simulink library "SingleWorkstationModelLibrary"  (R2014a)
settings: Solver=ode45  StartTime=0.0  StopTime=10.0  RelTol=1e-3
undefined symbols (not defined in the file or in its folder): se_randomizeseeds
(part 1 of 3)
settings Model: Creator=AnotherUser  LastModifiedBy=AnotherUser

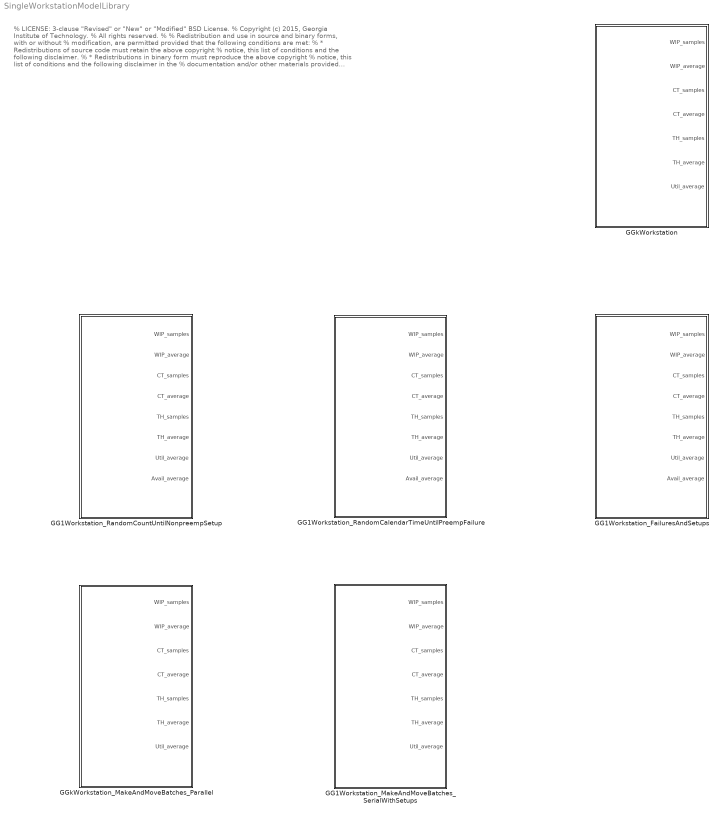
== system SingleWorkstationModelLibrary ==
  note: % LICENSE: 3-clause "Revised" or "New" or "Modified" BSD License.
      | % Copyright (c) 2015, Georgia Institute of Technology.
      | % All rights reserved.
      | %
      | % Redistribution and use in source and binary forms, with or without
      | % modification, are permitted provided that the following conditions are met:
      | % * Redistributions of source code must retain the above copyright
      | % notice, this list of conditions and the following disclaimer.
      | % * Redistributions in binary form must reproduce the above copyright
      | % notice, this list of conditions and the following disclaimer in the
      | % documentation and/or other materials provided with the distribution.
      | % * Neither the name of the Georgia Institute of Technology nor the
      | % names of its contributors may be used to endorse or promote products
      | % derived from this software without specific prior written permission.
      | %
      | % THIS SOFTWARE IS PROVIDED BY THE COPYRIGHT HOLDERS AND CONTRIBUTORS "AS IS" AND
      | % ANY EXPRESS OR IMPLIED WARRANTIES, INCLUDING, BUT NOT LIMITED TO, THE IMPLIED
      | % WARRANTIES OF MERCHANTABILITY AND FITNESS FOR A PARTICULAR PURPOSE ARE
      | % DISCLAIMED. IN NO EVENT SHALL THE GEORGIA INSTITUTE OF TECHNOLOGY BE LIABLE FOR
      | % ANY DIRECT, INDIRECT, INCIDENTAL, SPECIAL, EXEMPLARY, OR CONSEQUENTIAL DAMAGES
      | % (INCLUDING, BUT NOT LIMITED TO, PROCUREMENT OF SUBSTITUTE GOODS OR SERVICES;
      | % LOSS OF USE, DATA, OR PROFITS; OR BUSINESS INTERRUPTION) HOWEVER CAUSED AND
      | % ON ANY THEORY OF LIABILITY, WHETHER IN CONTRACT, STRICT LIABILITY, OR TORT
      | % (INCLUDING NEGLIGENCE OR OTHERWISE) ARISING IN ANY WAY OUT OF THE USE OF THIS
      | % SOFTWARE, EVEN IF ADVISED OF THE POSSIBILITY OF SUCH DAMAGE.
  GG1Workstation_FailuresAndSetups : Subsystem  InitFcn=se_randomizeseeds(gcs, 'Mode', 'All')
      settings: CopyFcn=set_param(gcb, 'LinkStatus', 'none');
  GG1Workstation_MakeAndMoveBatches_SerialWithSetups : Subsystem  InitFcn=se_randomizeseeds(gcs, 'Mode', 'All')
      settings: CopyFcn=set_param(gcb, 'LinkStatus', 'none');
  GG1Workstation_RandomCalendarTimeUntilPreempFailure : Subsystem  InitFcn=se_randomizeseeds(gcs, 'Mode', 'All')
      settings: CopyFcn=set_param(gcb, 'LinkStatus', 'none');
  GG1Workstation_RandomCountUntilNonpreempSetup : Subsystem  InitFcn=se_randomizeseeds(gcs, 'Mode', 'All')
      settings: CopyFcn=set_param(gcb, 'LinkStatus', 'none');
  GGkWorkstation : Subsystem  InitFcn=se_randomizeseeds(gcs, 'Mode', 'All')
      settings: CopyFcn=set_param(gcb, 'LinkStatus', 'none');
  GGkWorkstation_MakeAndMoveBatches_Parallel : Subsystem  InitFcn=se_randomizeseeds(gcs, 'Mode', 'All')
      settings: CopyFcn=set_param(gcb, 'LinkStatus', 'none');

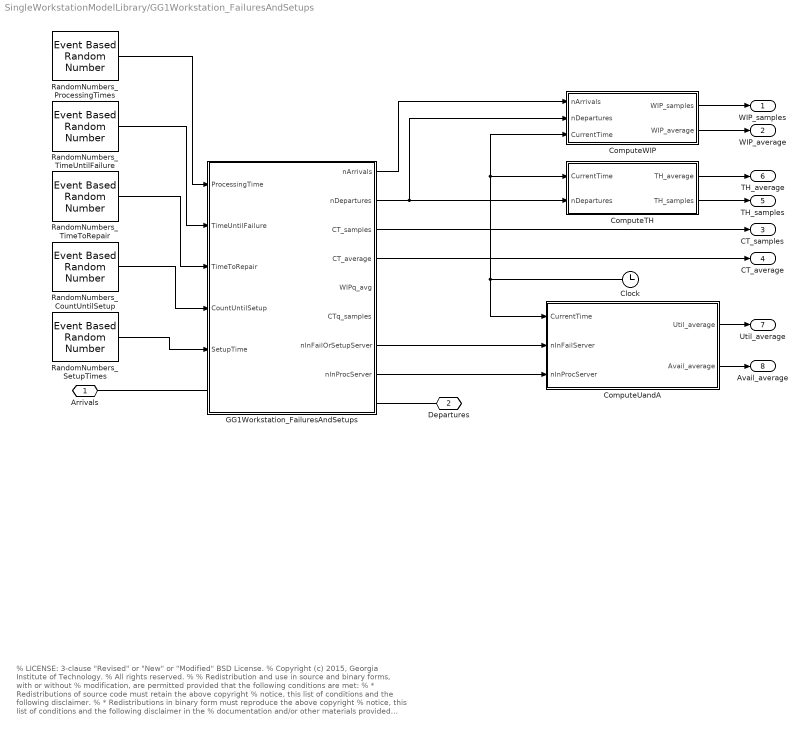
== system SingleWorkstationModelLibrary/GG1Workstation_FailuresAndSetups ==
  note: % LICENSE: 3-clause "Revised" or "New" or "Modified" BSD License.
      | % Copyright (c) 2015, Georgia Institute of Technology.
      | % All rights reserved.
      | %
      | % Redistribution and use in source and binary forms, with or without
      | % modification, are permitted provided that the following conditions are met:
      | % * Redistributions of source code must retain the above copyright
      | % notice, this list of conditions and the following disclaimer.
      | % * Redistributions in binary form must reproduce the above copyright
      | % notice, this list of conditions and the following disclaimer in the
      | % documentation and/or other materials provided with the distribution.
      | % * Neither the name of the Georgia Institute of Technology nor the
      | % names of its contributors may be used to endorse or promote products
      | % derived from this software without specific prior written permission.
      | %
      | % THIS SOFTWARE IS PROVIDED BY THE COPYRIGHT HOLDERS AND CONTRIBUTORS "AS IS" AND
      | % ANY EXPRESS OR IMPLIED WARRANTIES, INCLUDING, BUT NOT LIMITED TO, THE IMPLIED
      | % WARRANTIES OF MERCHANTABILITY AND FITNESS FOR A PARTICULAR PURPOSE ARE
      | % DISCLAIMED. IN NO EVENT SHALL THE GEORGIA INSTITUTE OF TECHNOLOGY BE LIABLE FOR
      | % ANY DIRECT, INDIRECT, INCIDENTAL, SPECIAL, EXEMPLARY, OR CONSEQUENTIAL DAMAGES
      | % (INCLUDING, BUT NOT LIMITED TO, PROCUREMENT OF SUBSTITUTE GOODS OR SERVICES;
      | % LOSS OF USE, DATA, OR PROFITS; OR BUSINESS INTERRUPTION) HOWEVER CAUSED AND
      | % ON ANY THEORY OF LIABILITY, WHETHER IN CONTRACT, STRICT LIABILITY, OR TORT
      | % (INCLUDING NEGLIGENCE OR OTHERWISE) ARISING IN ANY WAY OUT OF THE USE OF THIS
      | % SOFTWARE, EVEN IF ADVISED OF THE POSSIBILITY OF SUCH DAMAGE.
  Clock : Clock
  ComputeTH : Subsystem
  ComputeUandA : Subsystem
  ComputeWIP : Subsystem
  GG1Workstation_FailuresAndSetups : Subsystem  mask{Capacity=Inf}
      mask prompts: Capacity "Queue Capacity"
      mask TypeOptions Capacity: FIFOQueue/Capacity
      mask DialogControl DescTextVar Prompt: GG1 Workstation, with a random count of entities serviced until a setup, and random setup times.  Setups are functionally equivalent to any non-preemptive (e.g. non-interrupting) downtime, for example preventative maintenance.
  RandomNumbers_CountUntilSetup : EventBasedRandomNumber  meanExp=100  minUnif=40  maxUnif=40  pOneBern=40  pSuccessBino=40  numTrialBino=40  minTri=10  maxTri=10  modeTri=10  scaleGam=166.6667  shapeGam=0.72  meanNorm=200  stdNorm=eps  pSuccessGeo=40  meanPoiss=40  thresholdLogn=40  scaleLogn=40  shapeLogn=40  thresholdLogl=40  scaleLogl=40  minBeta=40  maxBeta=40  shape1Beta=40  shape2Beta=40  minUnid=40  maxUnid=40  numValueUnid=40  thresholdWbl=40  scaleWbl=40  shapeWbl=40  valueVecCont=40  cdfVecCont=40  valueVecDisc=40  probVecDisc=40  Seed=13103
  RandomNumbers_ProcessingTimes : EventBasedRandomNumber  meanExp=75  minUnif=40  maxUnif=40  pOneBern=40  pSuccessBino=40  numTrialBino=40  minTri=40  maxTri=40  modeTri=40  thresholdGam=40  scaleGam=40  shapeGam=40  meanNorm=50  stdNorm=eps  pSuccessGeo=40  meanPoiss=40  thresholdLogn=40  scaleLogn=40  shapeLogn=40  thresholdLogl=40  scaleLogl=40  minBeta=40  maxBeta=40  shape1Beta=40  shape2Beta=40  minUnid=40  maxUnid=40  numValueUnid=40  thresholdWbl=40  scaleWbl=40  shapeWbl=40  valueVecCont=40  cdfVecCont=40  valueVecDisc=40  probVecDisc=40  Seed=16319
  RandomNumbers_SetupTimes : EventBasedRandomNumber  meanExp=400  minUnif=40  maxUnif=40  pOneBern=40  pSuccessBino=40  numTrialBino=40  minTri=38  maxTri=38  modeTri=38  scaleGam=20  meanNorm=200  stdNorm=eps  pSuccessGeo=40  meanPoiss=40  thresholdLogn=40  scaleLogn=40  shapeLogn=40  thresholdLogl=40  scaleLogl=40  minBeta=40  maxBeta=40  shape1Beta=40  shape2Beta=40  minUnid=40  maxUnid=40  numValueUnid=40  thresholdWbl=40  scaleWbl=40  shapeWbl=40  valueVecCont=40  cdfVecCont=40  probVecDisc=[0 1]  Seed=19536
  RandomNumbers_TimeToRepair : EventBasedRandomNumber  meanExp=400  minUnif=40  maxUnif=40  pOneBern=40  pSuccessBino=40  numTrialBino=40  minTri=38  maxTri=38  modeTri=38  scaleGam=20  meanNorm=400  stdNorm=eps  pSuccessGeo=40  meanPoiss=40  thresholdLogn=40  scaleLogn=40  shapeLogn=40  thresholdLogl=40  scaleLogl=40  minBeta=40  maxBeta=40  shape1Beta=40  shape2Beta=40  minUnid=40  maxUnid=40  numValueUnid=40  thresholdWbl=40  scaleWbl=40  shapeWbl=40  valueVecCont=40  cdfVecCont=40  probVecDisc=[0 1]  Seed=22753
  RandomNumbers_TimeUntilFailure : EventBasedRandomNumber  meanExp=2500  minUnif=40  maxUnif=40  pOneBern=40  pSuccessBino=40  numTrialBino=40  minTri=114  maxTri=114  modeTri=114  scaleGam=166.6667  shapeGam=0.72  meanNorm=2000  stdNorm=eps  pSuccessGeo=40  meanPoiss=40  thresholdLogn=40  scaleLogn=40  shapeLogn=40  thresholdLogl=40  scaleLogl=40  minBeta=40  maxBeta=40  shape1Beta=40  shape2Beta=40  minUnid=40  maxUnid=40  numValueUnid=40  thresholdWbl=40  scaleWbl=40  shapeWbl=40  valueVecCont=40  cdfVecCont=40  valueVecDisc=40  probVecDisc=40  Seed=25970
  Arrivals : PMIOPort  Port=1  Side=Left
  Departures : PMIOPort  Port=2  Side=Right
  WIP_samples : Outport
  WIP_average : Outport  Port=2
  CT_samples : Outport  Port=3
  CT_average : Outport  Port=4
  TH_samples : Outport  Port=5
  TH_average : Outport  Port=6
  Util_average : Outport  Port=7
  Avail_average : Outport  Port=8
  wires:
  RandomNumbers_ProcessingTimes/1 -> GG1Workstation_FailuresAndSetups/1(ProcessingTime)
  GG1Workstation_FailuresAndSetups/2(nDepartures) -> ComputeWIP/2(nDepartures), ComputeTH/2(nDepartures)
  GG1Workstation_FailuresAndSetups/3(CT_samples) -> CT_samples/1
  GG1Workstation_FailuresAndSetups/4(CT_average) -> CT_average/1
  ComputeWIP/1(WIP_samples) -> WIP_samples/1
  ComputeWIP/2(WIP_average) -> WIP_average/1
  GG1Workstation_FailuresAndSetups/1(nArrivals) -> ComputeWIP/1(nArrivals)
  Clock/1 -> ComputeWIP/3(CurrentTime), ComputeTH/1(CurrentTime), ComputeUandA/1(CurrentTime)
  ComputeTH/1(TH_average) -> TH_average/1
  ComputeTH/2(TH_samples) -> TH_samples/1
  RandomNumbers_TimeUntilFailure/1 -> GG1Workstation_FailuresAndSetups/2(TimeUntilFailure)
  RandomNumbers_TimeToRepair/1 -> GG1Workstation_FailuresAndSetups/3(TimeToRepair)
  RandomNumbers_CountUntilSetup/1 -> GG1Workstation_FailuresAndSetups/4(CountUntilSetup)
  RandomNumbers_SetupTimes/1 -> GG1Workstation_FailuresAndSetups/5(SetupTime)
  GG1Workstation_FailuresAndSetups/7(nInFailOrSetupServer) -> ComputeUandA/2(nInFailServer)
  GG1Workstation_FailuresAndSetups/8(nInProcServer) -> ComputeUandA/3(nInProcServer)
  ComputeUandA/1(Util_average) -> Util_average/1
  ComputeUandA/2(Avail_average) -> Avail_average/1
  connections:
  GG1Workstation_FailuresAndSetups/RConn1 -- Departures/RConn1
  Arrivals/RConn1 -- GG1Workstation_FailuresAndSetups/LConn1

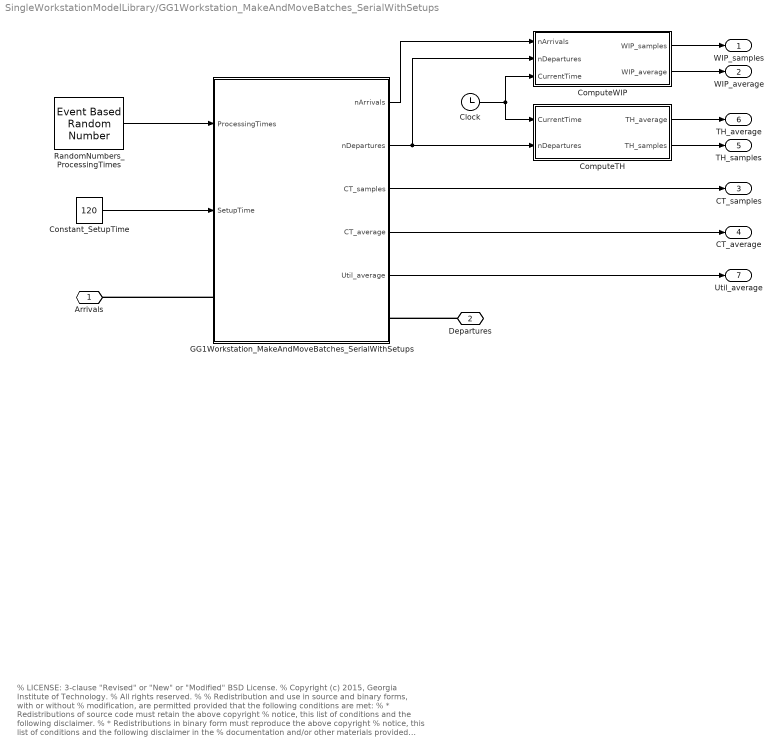
== system SingleWorkstationModelLibrary/GG1Workstation_MakeAndMoveBatches_SerialWithSetups ==
  note: % LICENSE: 3-clause "Revised" or "New" or "Modified" BSD License.
      | % Copyright (c) 2015, Georgia Institute of Technology.
      | % All rights reserved.
      | %
      | % Redistribution and use in source and binary forms, with or without
      | % modification, are permitted provided that the following conditions are met:
      | % * Redistributions of source code must retain the above copyright
      | % notice, this list of conditions and the following disclaimer.
      | % * Redistributions in binary form must reproduce the above copyright
      | % notice, this list of conditions and the following disclaimer in the
      | % documentation and/or other materials provided with the distribution.
      | % * Neither the name of the Georgia Institute of Technology nor the
      | % names of its contributors may be used to endorse or promote products
      | % derived from this software without specific prior written permission.
      | %
      | % THIS SOFTWARE IS PROVIDED BY THE COPYRIGHT HOLDERS AND CONTRIBUTORS "AS IS" AND
      | % ANY EXPRESS OR IMPLIED WARRANTIES, INCLUDING, BUT NOT LIMITED TO, THE IMPLIED
      | % WARRANTIES OF MERCHANTABILITY AND FITNESS FOR A PARTICULAR PURPOSE ARE
      | % DISCLAIMED. IN NO EVENT SHALL THE GEORGIA INSTITUTE OF TECHNOLOGY BE LIABLE FOR
      | % ANY DIRECT, INDIRECT, INCIDENTAL, SPECIAL, EXEMPLARY, OR CONSEQUENTIAL DAMAGES
      | % (INCLUDING, BUT NOT LIMITED TO, PROCUREMENT OF SUBSTITUTE GOODS OR SERVICES;
      | % LOSS OF USE, DATA, OR PROFITS; OR BUSINESS INTERRUPTION) HOWEVER CAUSED AND
      | % ON ANY THEORY OF LIABILITY, WHETHER IN CONTRACT, STRICT LIABILITY, OR TORT
      | % (INCLUDING NEGLIGENCE OR OTHERWISE) ARISING IN ANY WAY OUT OF THE USE OF THIS
      | % SOFTWARE, EVEN IF ADVISED OF THE POSSIBILITY OF SUCH DAMAGE.
  Clock : Clock
  ComputeTH : Subsystem
  ComputeWIP : Subsystem
  Constant_SetupTime : Constant  Value=120
  GG1Workstation_MakeAndMoveBatches_SerialWithSetups : Subsystem  mask{MakeBatchSize=10, MoveBatchSize=1}
      mask prompts: MakeBatchSize "Make (a.k.a. Process) Batch Size:"; MoveBatchSize "Move (a.k.a. Transfer) Batch Size"
      mask Callback MakeBatchSize:
      | %% Capture pre-existing base workspace variables, to cleanup when done
      | preExistingVars = who;
      | 
      | 
      | %% MakeBatchSize is defined as a mask parameter
      | batchSizeStr = get_param(gcbh, 'MakeBatchSize');
      | batchSizeInt = int32(str2double(batchSizeStr));  %Enforce integer
      | if batchSizeInt < 1  %str2double returns NaN for non-numerical input, and int32 returns 0 for NaN
      |     error('Invalid input for MakeBatchSize');
      | end
      | set_param(gcbh, 'MakeBatchSize', num2str(batchSizeInt));  %Correct any non-integer value
      | 
      | 
      | %% Get paths of OutputSwitch, EntityCombiner, EntitySplitter, and PathCombiner
      | singleWksPath = [gcs '/' get(gcbh,'Name')];
      | outputSwitchPath = [singleWksPath '/MakeBatchOutputSwitch'];
      | entityCombinerPath = [singleWksPath '/MakeBatchEntityCombiner'];
      | entitySplitterPath = [singleWksPath '/MakeBatchEntitySplitter'];
      | pathCombinerPath = [singleWksPath '/MakeBatchPathCombiner'];
      | 
      | 
      | %% NEW
      | constantPath = [singleWksPath '/Constant_MakeBatchSize'];
      | set_param(constantPath, 'Value', num2str(batchSizeInt));
      | 
      | 
      | %% Unsure if needed:  Disable model library link to enable editing
      | %set_param(singleWksPath, 'LinkStatus', 'inactive');
      | 
      | 
      | %% Delete existing queues and connections
      | phOutputSwitch = get_param(outputSwitchPath, 'PortHandles');
      | phOutputSwitch = phOutputSwitch.RConn;
      | phEntityCombiner = get_param(entityCombinerPath, 'PortHandles');
      | phEntityCombiner = phEntityCombiner.LConn;
      | phEntitySplitter = get_param(entitySplitterPath, 'PortHandles');
      | phEntitySplitter = phEntitySplitter.RConn;
      | phPathCombiner = get_param(pathCombinerPath, 'PortHandles');
      | phPathCombiner = phPathCombiner.LConn;
      | 
      | 
      | %Delete existing queues
      | oldBatchSize = get_param(outputSwitchPath, 'NumberOutputPorts');
      | queueNamesBeginWith = 'MakeBatchQ';  %Hard-codes a particular naming scheme
      | singleWksBlockList = get(gcbh, 'Blocks');
      | ECQueueMatches = strncmpi(queueNamesBeginWith, singleWksBlockList, length(queueNamesBeginWith));
      | ECQueueNames = singleWksBlockList(ECQueueMatches);
      | if ~isempty(ECQueueNames)
      |     for mmmmm = 1 : length(ECQueueNames)
      |         queuePath = [singleWksPath '/' ECQueueNames{mmmmm}];
      |         queueHandle = get_param(queuePath, 'Handle');
      |         delete(queueHandle);
      |     end
      | end
      | 
      | %Delete the lines
      | for iiiii = 1 : str2double(oldBatchSize)
      |     phOutputSwitchPos = get_param(phOutputSwitch(iiiii), 'Position');
      |     try delete_line(singleWksPath, phOutputSwitchPos); catch, end  %Fail silently
      |     phEntityCombinerPos = get_param(phEntityCombiner(iiiii), 'Position');
      |     try delete_line(singleWksPath, phEntityCombinerPos); catch, end  %Fail silently
      |     phEntitySplitterPos = get_param(phEntitySplitter(iiiii), 'Position');
      |     try delete_line(singleWksPath, phEntitySplitterPos); catch, end  %Fail silently
      | 	phPathCombinerPos = get_param(phPathCombiner(iiiii), 'Position');
      | 	try delete_line(singleWksPath, phPathCombinerPos); catch, end  %Fail silently
      | end
      | 
      | 
      | %% Set new number of ports
      | set_param(outputSwitchPath, 'NumberOutputPorts', batchSizeStr);
      | set_param(entityCombinerPath, 'NumberInputPorts', batchSizeStr);
      | set_param(entitySplitterPath, 'NumberOutputPorts', batchSizeStr);
      | set_param(pathCombinerPath, 'NumberInputPorts', batchSizeStr);
      | 
      | 
      | %% Add queues and connectors
      | phOutputSwitch = get_param(outputSwitchPath, 'PortHandles');
      | phOutputSwitch = phOutputSwitch.RConn;
      | phEntityCombiner = get_param(entityCombinerPath, 'PortHandles');
      | phEntityCombiner = phEntityCombiner.LConn;
      | phEntitySplitter = get_param(entitySplitterPath, 'PortHandles');
      | phEntitySplitter = phEntitySplitter.RConn;
      | phPathCombiner = get_param(pathCombinerPath, 'PortHandles');
      | phPathCombiner = phPathCombiner.LConn;
      | 
      | queueLength = 80;
      | queueHeight = 20;
      | xOffset = 130;
      | prevBlockPos1 = get_param(outputSwitchPath, 'Position');
      | prevBlockPos2 = get_param(entitySplitterPath, 'Position');
      | prevBlockHeight1 = prevBlockPos1(4)-prevBlockPos1(2);
      | prevBlockHeight2 = prevBlockPos2(4)-prevBlockPos2(2);
      | yIncrement1 = prevBlockHeight1 / batchSizeInt;
      | yIncrement2 = prevBlockHeight2 / batchSizeInt;
      | for jjjjj = 1 : batchSizeInt
      | 	%%%%%%%%%%
      | 	%OutputSwitch to EntityCombiner
      |     queuePath = [singleWksPath '/' queueNamesBeginWith num2str(jjjjj) 'a'];
      |     queueHandle = add_block('built-in/FIFOQueue', queuePath);
      |     set_param(queueHandle, 'Capacity', 'Inf');  %Shouldn't be needed, but a good default
      | 
      |     left = prevBlockPos1(1)+xOffset;
      |     top = double( prevBlockPos1(2)+(jjjjj-1)*yIncrement1 );
      |     right = prevBlockPos1(1)+xOffset+queueLength;
      |     bottom = double( prevBlockPos1(2)+(jjjjj-1)*yIncrement1+queueHeight );
      |     p = [left top right bottom];
      |     set_param(queueHandle, 'Position', p);  %Need a vector of doubles (not int32)
      | 
      |     QueuePortHandles = get_param(queueHandle, 'PortHandles');
      |     %Line from OutputSwitch to Queue
      |     OutputSwitchOutPortPos = get_param(phOutputSwitch(jjjjj), 'Position');
      |     QueueInPortPos = get_param(QueuePortHandles.LConn, 'Position');
      |     add_line(singleWksPath, [OutputSwitchOutPortPos; QueueInPortPos]);
      |     %Line from Queue to EntityCombiner
      |     QueueOutPortPos = get_param(QueuePortHandles.RConn, 'Position');
      |     EntityCombinerInPortPos = get_param(phEntityCombiner(jjjjj), 'Position');
      |     add_line(singleWksPath, [QueueOutPortPos; EntityCombinerInPortPos]);
      | 
      | 	%%%%%%%%%%
      | 	%EntitySplitter to PathCombiner
      | 	queuePath = [singleWksPath '/' queueNamesBeginWith num2str(jjjjj) 'b'];
      |     queueHandle = add_block('built-in/FIFOQueue', queuePath);
      |     set_param(queueHandle, 'Capacity', num2str(1));  %Second set of queues have capacity 1
      | 
      |     left = prevBlockPos2(1)+xOffset;
      |     top = double( prevBlockPos2(2)+(jjjjj-1)*yIncrement2 );
      |     right = prevBlockPos2(1)+xOffset+queueLength;
      |     bottom = double( prevBlockPos2(2)+(jjjjj-1)*yIncrement2+queueHeight );
      |     p = [left top right bottom];
      |     set_param(queueHandle, 'Position', p);  %Need a vector of doubles (not int32)
      | 
      |     QueuePortHandles = get_param(queueHandle, 'PortHandles');
      |     %Line from OutputSwitch to Queue
      |     EntitySplitterOutPortPos = get_param(phEntitySplitter(jjjjj), 'Position');
      |     QueueInPortPos = get_param(QueuePortHandles.LConn, 'Position');
      |     add_line(singleWksPath, [EntitySplitterOutPortPos; QueueInPortPos]);
      |     %Line from Queue to EntityCombiner
      |     QueueOutPortPos = get_param(QueuePortHandles.RConn, 'Position');
      |     PathCombinerInPortPos = get_param(phPathCombiner(jjjjj), 'Position');
      |     add_line(singleWksPath, [QueueOutPortPos; PathCombinerInPortPos ]);
      | end
      | 
      | 
      | %% Cleanup, because mask callback executes in base workspace
      | clearvars('-except', preExistingVars{:});
      mask Callback MoveBatchSize:
      | %% Capture pre-existing base workspace variables, to cleanup when done
      | preExistingVars = who;
      | 
      | 
      | %% MoveBatchSize is defined as a mask parameter
      | batchSizeStr = get_param(gcbh, 'MoveBatchSize');
      | batchSizeInt = int32(str2double(batchSizeStr));  %Enforce integer
      | if batchSizeInt < 1  %str2double returns NaN for non-numerical input, and int32 returns 0 for NaN
      |     error('Invalid input for MoveBatchSize');
      | end
      | set_param(gcbh, 'MoveBatchSize', num2str(batchSizeInt));  %Correct any non-integer value
      | 
      | 
      | %% Get paths of OutputSwitch, EntityCombiner, EntitySplitter, and PathCombiner
      | singleWksPath = [gcs '/' get(gcbh,'Name')];
      | outputSwitchPath = [singleWksPath '/MoveBatchOutputSwitch'];
      | entityCombinerPath = [singleWksPath '/MoveBatchEntityCombiner'];
      | entitySplitterPath = [singleWksPath '/MoveBatchEntitySplitter'];
      | pathCombinerPath = [singleWksPath '/MoveBatchPathCombiner'];
      | 
      | 
      | %% Unsure if needed:  Disable model library link to enable editing
      | %set_param(singleWksPath, 'LinkStatus', 'inactive');
      | 
      | 
      | %% Delete existing queues and connections
      | phOutputSwitch = get_param(outputSwitchPath, 'PortHandles');
      | phOutputSwitch = phOutputSwitch.RConn;
      | phEntityCombiner = get_param(entityCombinerPath, 'PortHandles');
      | phEntityCombiner = phEntityCombiner.LConn;
      | phEntitySplitter = get_param(entitySplitterPath, 'PortHandles');
      | phEntitySplitter = phEntitySplitter.RConn;
      | 
      | %Delete existing queues
      | oldBatchSize = get_param(outputSwitchPath, 'NumberOutputPorts');
      | queueNamesBeginWith = 'MoveBatchQ';  %Hard-codes a particular naming scheme
      | singleWksBlockList = get(gcbh, 'Blocks');
      | ECQueueMatches = strncmpi(queueNamesBeginWith, singleWksBlockList, length(queueNamesBeginWith));
      | ECQueueNames = singleWksBlockList(ECQueueMatches);
      | if ~isempty(ECQueueNames)
      |     for mmmmm = 1 : length(ECQueueNames)
      |         queuePath = [singleWksPath '/' ECQueueNames{mmmmm}];
      |         queueHandle = get_param(queuePath, 'Handle');
      |         delete(queueHandle);
      |     end
      | end
      | 
      | %Delete the lines
      | for iiiii = 1 : str2double(oldBatchSize)
      |     phOutputSwitchPos = get_param(phOutputSwitch(iiiii), 'Position');
      |     try delete_line(singleWksPath, phOutputSwitchPos); catch, end  %Fail silently
      |     phEntityCombinerPos = get_param(phEntityCombiner(iiiii), 'Position');
      |     try delete_line(singleWksPath, phEntityCombinerPos); catch, end  %Fail silently
      |     phEntitySplitterPos = get_param(phEntitySplitter(iiiii), 'Position');
      |     try delete_line(singleWksPath, phEntitySplitterPos); catch, end  %Fail silently
      | end
      | 
      | 
      | %% Set new number of ports
      | set_param(outputSwitchPath, 'NumberOutputPorts', batchSizeStr);
      | set_param(entityCombinerPath, 'NumberInputPorts', batchSizeStr);
      | set_param(entitySplitterPath, 'NumberOutputPorts', batchSizeStr);
      | set_param(pathCombinerPath, 'NumberInputPorts', batchSizeStr);
      | 
      | 
      | %% Add EntityCombiner input queues, plus connections between OutputSwitch and EntityCombiner
      | phOutputSwitch = get_param(outputSwitchPath, 'PortHandles');
      | phOutputSwitch = phOutputSwitch.RConn;
      | phEntityCombiner = get_param(entityCombinerPath, 'PortHandles');
      | phEntityCombiner = phEntityCombiner.LConn;
      | phEntitySplitter = get_param(entitySplitterPath, 'PortHandles');
      | phEntitySplitter = phEntitySplitter.RConn;
      | phPathCombiner = get_param(pathCombinerPath, 'PortHandles');
      | phPathCombiner = phPathCombiner.LConn;
      | 
      | queueLength = 80;
      | queueHeight = 20;
      | xOffset = 130;
      | prevBlockPos = get_param(outputSwitchPath, 'Position');
      | prevBlockHeight = prevBlockPos(4)-prevBlockPos(2);
      | yIncrement = prevBlockHeight / batchSizeInt;
      | for jjjjj = 1 : batchSizeInt
      |     queuePath = [singleWksPath '/' queueNamesBeginWith num2str(jjjjj)];
      |     queueHandle = add_block('built-in/FIFOQueue', queuePath);
      |     set_param(queueHandle, 'Capacity', '1');
      | 
      | 	left = prevBlockPos(1)+xOffset;
      |     top = double( prevBlockPos(2)+(jjjjj-1)*yIncrement );
      |     right = prevBlockPos(1)+xOffset+queueLength;
      |     bottom = double( prevBlockPos(2)+(jjjjj-1)*yIncrement+queueHeight );
      |     p = [left top right bottom];
      |     set_param(queueHandle, 'Position', p);  %Need a vector of doubles (not int32)
      | 
      |     QueuePortHandles = get_param(queueHandle, 'PortHandles');
      |     %Line from OutputSwitch to Queue
      |     OutputSwitchOutPortPos = get_param(phOutputSwitch(jjjjj), 'Position');
      |     QueueInPortPos = get_param(QueuePortHandles.LConn, 'Position');
      |     add_line(singleWksPath, [OutputSwitchOutPortPos; QueueInPortPos]);
      |     %Line from Queue to EntityCombiner
      |     QueueOutPortPos = get_param(QueuePortHandles.RConn, 'Position');
      |     EntityCombinerInPortPos = get_param(phEntityCombiner(jjjjj), 'Position');
      |     add_line(singleWksPath, [QueueOutPortPos; EntityCombinerInPortPos]);
      | end
      | 
      | 
      | %% Add connections between EntitySplitter and PathCombiner
      | for kkkkk = 1 : batchSizeInt
      |     phEntitySplitterPos = get_param(phEntitySplitter(kkkkk), 'Position');
      |     phPathCombinerPos = get_param(phPathCombiner(kkkkk), 'Position');
      |     add_line(singleWksPath, [phEntitySplitterPos; phPathCombinerPos]);
      | end
      | 
      | 
      | %% Cleanup, because mask callback executes in base workspace
      | clearvars('-except', preExistingVars{:});
      mask DialogControl DescTextVar Prompt: GGk Workstation with Make and Move Batches.  This model implements serial batch processing, meaning Processing Time is for each element in a make (a.k.a. process) batch.  Tokens are output only after a full move (a.k.a. transfer) batch is assembled, and are output individually (as individual entities, not as a batch entity).
  RandomNumbers_ProcessingTimes : EventBasedRandomNumber  Distribution=Gaussian (normal)  meanExp=10  minUnif=40  maxUnif=40  pOneBern=40  pSuccessBino=40  numTrialBino=40  minTri=40  maxTri=40  modeTri=40  thresholdGam=40  scaleGam=40  shapeGam=40  meanNorm=10  stdNorm=eps  pSuccessGeo=40  meanPoiss=40  thresholdLogn=40  scaleLogn=40  shapeLogn=40  thresholdLogl=40  scaleLogl=40  minBeta=40  maxBeta=40  shape1Beta=40  shape2Beta=40  minUnid=40  maxUnid=40  numValueUnid=40  thresholdWbl=40  scaleWbl=40  shapeWbl=40  valueVecCont=40  cdfVecCont=40  valueVecDisc=40  probVecDisc=40  Seed=54923
  Arrivals : PMIOPort  Port=1  Side=Left
  Departures : PMIOPort  Port=2  Side=Right
  WIP_samples : Outport
  WIP_average : Outport  Port=2
  CT_samples : Outport  Port=3
  CT_average : Outport  Port=4
  TH_samples : Outport  Port=5
  TH_average : Outport  Port=6
  Util_average : Outport  Port=7
  wires:
  RandomNumbers_ProcessingTimes/1 -> GG1Workstation_MakeAndMoveBatches_SerialWithSetups/1(ProcessingTimes)
  GG1Workstation_MakeAndMoveBatches_SerialWithSetups/2(nDepartures) -> ComputeWIP/2(nDepartures), ComputeTH/2(nDepartures)
  GG1Workstation_MakeAndMoveBatches_SerialWithSetups/3(CT_samples) -> CT_samples/1
  GG1Workstation_MakeAndMoveBatches_SerialWithSetups/4(CT_average) -> CT_average/1
  ComputeWIP/1(WIP_samples) -> WIP_samples/1
  ComputeWIP/2(WIP_average) -> WIP_average/1
  GG1Workstation_MakeAndMoveBatches_SerialWithSetups/1(nArrivals) -> ComputeWIP/1(nArrivals)
  Clock/1 -> ComputeTH/1(CurrentTime), ComputeWIP/3(CurrentTime)
  ComputeTH/1(TH_average) -> TH_average/1
  ComputeTH/2(TH_samples) -> TH_samples/1
  GG1Workstation_MakeAndMoveBatches_SerialWithSetups/5(Util_average) -> Util_average/1
  Constant_SetupTime/1 -> GG1Workstation_MakeAndMoveBatches_SerialWithSetups/2(SetupTime)
  connections:
  Departures/RConn1 -- GG1Workstation_MakeAndMoveBatches_SerialWithSetups/RConn1
  GG1Workstation_MakeAndMoveBatches_SerialWithSetups/LConn1 -- Arrivals/RConn1

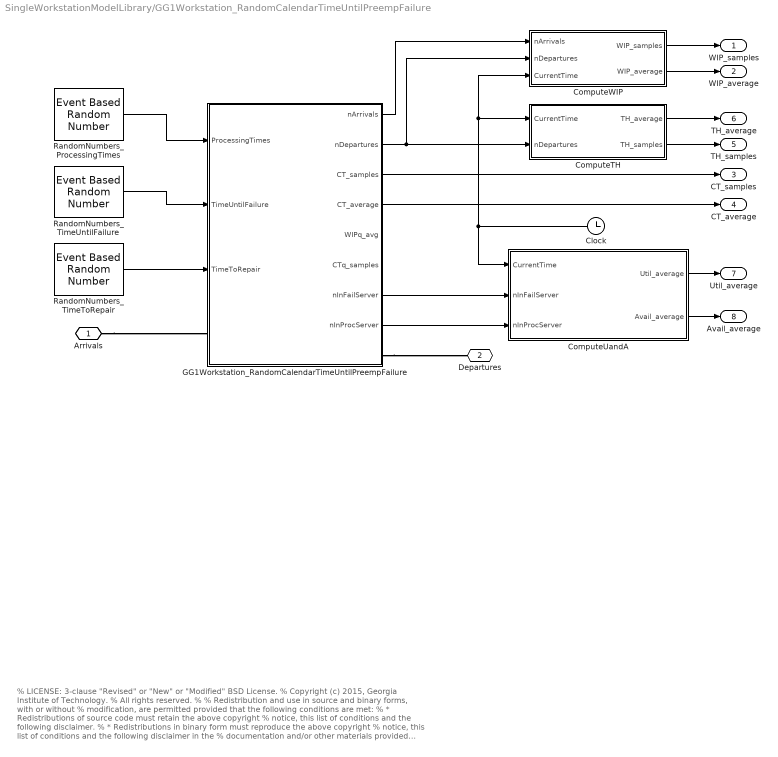
== system SingleWorkstationModelLibrary/GG1Workstation_RandomCalendarTimeUntilPreempFailure ==
  note: % LICENSE: 3-clause "Revised" or "New" or "Modified" BSD License.
      | % Copyright (c) 2015, Georgia Institute of Technology.
      | % All rights reserved.
      | %
      | % Redistribution and use in source and binary forms, with or without
      | % modification, are permitted provided that the following conditions are met:
      | % * Redistributions of source code must retain the above copyright
      | % notice, this list of conditions and the following disclaimer.
      | % * Redistributions in binary form must reproduce the above copyright
      | % notice, this list of conditions and the following disclaimer in the
      | % documentation and/or other materials provided with the distribution.
      | % * Neither the name of the Georgia Institute of Technology nor the
      | % names of its contributors may be used to endorse or promote products
      | % derived from this software without specific prior written permission.
      | %
      | % THIS SOFTWARE IS PROVIDED BY THE COPYRIGHT HOLDERS AND CONTRIBUTORS "AS IS" AND
      | % ANY EXPRESS OR IMPLIED WARRANTIES, INCLUDING, BUT NOT LIMITED TO, THE IMPLIED
      | % WARRANTIES OF MERCHANTABILITY AND FITNESS FOR A PARTICULAR PURPOSE ARE
      | % DISCLAIMED. IN NO EVENT SHALL THE GEORGIA INSTITUTE OF TECHNOLOGY BE LIABLE FOR
      | % ANY DIRECT, INDIRECT, INCIDENTAL, SPECIAL, EXEMPLARY, OR CONSEQUENTIAL DAMAGES
      | % (INCLUDING, BUT NOT LIMITED TO, PROCUREMENT OF SUBSTITUTE GOODS OR SERVICES;
      | % LOSS OF USE, DATA, OR PROFITS; OR BUSINESS INTERRUPTION) HOWEVER CAUSED AND
      | % ON ANY THEORY OF LIABILITY, WHETHER IN CONTRACT, STRICT LIABILITY, OR TORT
      | % (INCLUDING NEGLIGENCE OR OTHERWISE) ARISING IN ANY WAY OUT OF THE USE OF THIS
      | % SOFTWARE, EVEN IF ADVISED OF THE POSSIBILITY OF SUCH DAMAGE.
  Clock : Clock
  ComputeTH : Subsystem
  ComputeUandA : Subsystem
  ComputeWIP : Subsystem
  GG1Workstation_RandomCalendarTimeUntilPreempFailure : Subsystem  mask{Capacity=Inf}
      mask prompts: Capacity "Queue Capacity"
      mask TypeOptions Capacity: FIFOQueue/Capacity
      mask DialogControl DescTextVar Prompt: GG1 Workstation, with random time intervals until preemptive failure and random repair times.  Timing is consistent with Hopp & Spearman’s model, in that the time-until-failure clock stops during repair.
  RandomNumbers_ProcessingTimes : EventBasedRandomNumber  meanExp=80  minUnif=40  maxUnif=40  pOneBern=40  pSuccessBino=40  numTrialBino=40  minTri=40  maxTri=40  modeTri=40  thresholdGam=40  scaleGam=40  shapeGam=40  meanNorm=50  stdNorm=eps  pSuccessGeo=40  meanPoiss=40  thresholdLogn=40  scaleLogn=40  shapeLogn=40  thresholdLogl=40  scaleLogl=40  minBeta=40  maxBeta=40  shape1Beta=40  shape2Beta=40  minUnid=40  maxUnid=40  numValueUnid=40  thresholdWbl=40  scaleWbl=40  shapeWbl=40  valueVecCont=40  cdfVecCont=40  valueVecDisc=40  probVecDisc=40  Seed=62554
  RandomNumbers_TimeToRepair : EventBasedRandomNumber  meanExp=400  minUnif=40  maxUnif=40  pOneBern=40  pSuccessBino=40  numTrialBino=40  minTri=38  maxTri=38  modeTri=38  scaleGam=20  meanNorm=400  stdNorm=eps  pSuccessGeo=40  meanPoiss=40  thresholdLogn=40  scaleLogn=40  shapeLogn=40  thresholdLogl=40  scaleLogl=40  minBeta=40  maxBeta=40  shape1Beta=40  shape2Beta=40  minUnid=40  maxUnid=40  numValueUnid=40  thresholdWbl=40  scaleWbl=40  shapeWbl=40  valueVecCont=40  cdfVecCont=40  probVecDisc=[0 1]  Seed=235
  RandomNumbers_TimeUntilFailure : EventBasedRandomNumber  meanExp=2500  minUnif=40  maxUnif=40  pOneBern=40  pSuccessBino=40  numTrialBino=40  minTri=114  maxTri=114  modeTri=114  scaleGam=166.6667  shapeGam=0.72  meanNorm=2000  stdNorm=eps  pSuccessGeo=40  meanPoiss=40  thresholdLogn=40  scaleLogn=40  shapeLogn=40  thresholdLogl=40  scaleLogl=40  minBeta=40  maxBeta=40  shape1Beta=40  shape2Beta=40  minUnid=40  maxUnid=40  numValueUnid=40  thresholdWbl=40  scaleWbl=40  shapeWbl=40  valueVecCont=40  cdfVecCont=40  valueVecDisc=40  probVecDisc=40  Seed=3452
  Arrivals : PMIOPort  Port=1  Side=Left
  Departures : PMIOPort  Port=2  Side=Right
  WIP_samples : Outport
  WIP_average : Outport  Port=2
  CT_samples : Outport  Port=3
  CT_average : Outport  Port=4
  TH_samples : Outport  Port=5
  TH_average : Outport  Port=6
  Util_average : Outport  Port=7
  Avail_average : Outport  Port=8
  wires:
  RandomNumbers_ProcessingTimes/1 -> GG1Workstation_RandomCalendarTimeUntilPreempFailure/1(ProcessingTimes)
  GG1Workstation_RandomCalendarTimeUntilPreempFailure/2(nDepartures) -> ComputeTH/2(nDepartures), ComputeWIP/2(nDepartures)
  GG1Workstation_RandomCalendarTimeUntilPreempFailure/3(CT_samples) -> CT_samples/1
  GG1Workstation_RandomCalendarTimeUntilPreempFailure/4(CT_average) -> CT_average/1
  ComputeWIP/1(WIP_samples) -> WIP_samples/1
  ComputeWIP/2(WIP_average) -> WIP_average/1
  GG1Workstation_RandomCalendarTimeUntilPreempFailure/1(nArrivals) -> ComputeWIP/1(nArrivals)
  Clock/1 -> ComputeUandA/1(CurrentTime), ComputeTH/1(CurrentTime), ComputeWIP/3(CurrentTime)
  ComputeTH/1(TH_average) -> TH_average/1
  ComputeTH/2(TH_samples) -> TH_samples/1
  RandomNumbers_TimeUntilFailure/1 -> GG1Workstation_RandomCalendarTimeUntilPreempFailure/2(TimeUntilFailure)
  RandomNumbers_TimeToRepair/1 -> GG1Workstation_RandomCalendarTimeUntilPreempFailure/3(TimeToRepair)
  GG1Workstation_RandomCalendarTimeUntilPreempFailure/7(nInFailServer) -> ComputeUandA/2(nInFailServer)
  GG1Workstation_RandomCalendarTimeUntilPreempFailure/8(nInProcServer) -> ComputeUandA/3(nInProcServer)
  ComputeUandA/1(Util_average) -> Util_average/1
  ComputeUandA/2(Avail_average) -> Avail_average/1
  connections:
  GG1Workstation_RandomCalendarTimeUntilPreempFailure/RConn1 -- Departures/RConn1
  Arrivals/RConn1 -- GG1Workstation_RandomCalendarTimeUntilPreempFailure/LConn1

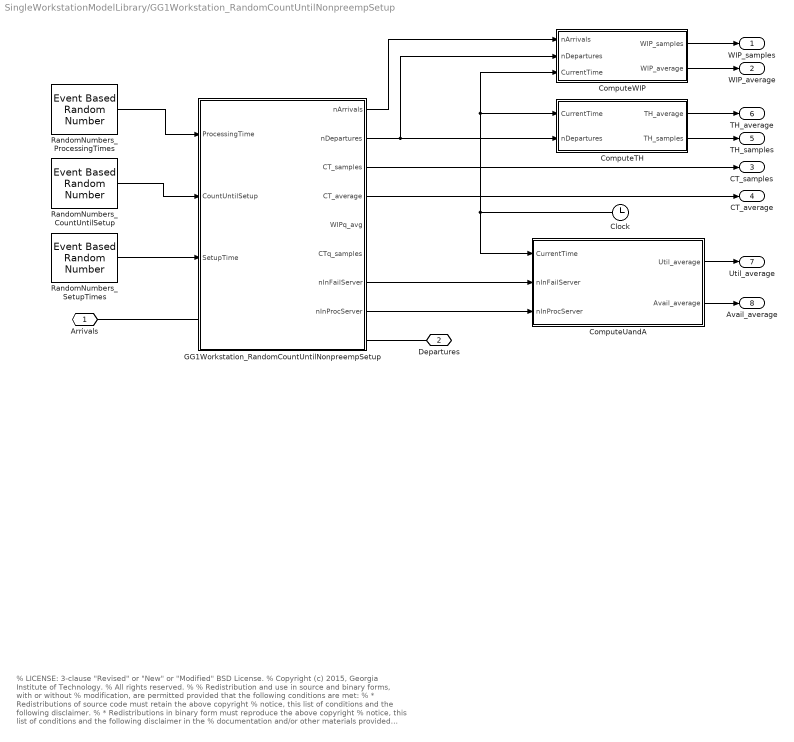
== system SingleWorkstationModelLibrary/GG1Workstation_RandomCountUntilNonpreempSetup ==
  note: % LICENSE: 3-clause "Revised" or "New" or "Modified" BSD License.
      | % Copyright (c) 2015, Georgia Institute of Technology.
      | % All rights reserved.
      | %
      | % Redistribution and use in source and binary forms, with or without
      | % modification, are permitted provided that the following conditions are met:
      | % * Redistributions of source code must retain the above copyright
      | % notice, this list of conditions and the following disclaimer.
      | % * Redistributions in binary form must reproduce the above copyright
      | % notice, this list of conditions and the following disclaimer in the
      | % documentation and/or other materials provided with the distribution.
      | % * Neither the name of the Georgia Institute of Technology nor the
      | % names of its contributors may be used to endorse or promote products
      | % derived from this software without specific prior written permission.
      | %
      | % THIS SOFTWARE IS PROVIDED BY THE COPYRIGHT HOLDERS AND CONTRIBUTORS "AS IS" AND
      | % ANY EXPRESS OR IMPLIED WARRANTIES, INCLUDING, BUT NOT LIMITED TO, THE IMPLIED
      | % WARRANTIES OF MERCHANTABILITY AND FITNESS FOR A PARTICULAR PURPOSE ARE
      | % DISCLAIMED. IN NO EVENT SHALL THE GEORGIA INSTITUTE OF TECHNOLOGY BE LIABLE FOR
      | % ANY DIRECT, INDIRECT, INCIDENTAL, SPECIAL, EXEMPLARY, OR CONSEQUENTIAL DAMAGES
      | % (INCLUDING, BUT NOT LIMITED TO, PROCUREMENT OF SUBSTITUTE GOODS OR SERVICES;
      | % LOSS OF USE, DATA, OR PROFITS; OR BUSINESS INTERRUPTION) HOWEVER CAUSED AND
      | % ON ANY THEORY OF LIABILITY, WHETHER IN CONTRACT, STRICT LIABILITY, OR TORT
      | % (INCLUDING NEGLIGENCE OR OTHERWISE) ARISING IN ANY WAY OUT OF THE USE OF THIS
      | % SOFTWARE, EVEN IF ADVISED OF THE POSSIBILITY OF SUCH DAMAGE.
  Clock : Clock
  ComputeTH : Subsystem
  ComputeUandA : Subsystem
  ComputeWIP : Subsystem
  GG1Workstation_RandomCountUntilNonpreempSetup : Subsystem  mask{Capacity=Inf}
      mask prompts: Capacity "Queue Capacity"
      mask TypeOptions Capacity: FIFOQueue/Capacity
      mask DialogControl DescTextVar Prompt: GG1 Workstation, with a random count of entities serviced until a setup, and random setup times.  Setups are functionally equivalent to any non-preemptive (e.g. non-interrupting) downtime, for example preventative maintenance.
  RandomNumbers_CountUntilSetup : EventBasedRandomNumber  meanExp=100  minUnif=40  maxUnif=40  pOneBern=40  pSuccessBino=40  numTrialBino=40  minTri=10  maxTri=10  modeTri=10  scaleGam=166.6667  shapeGam=0.72  meanNorm=200  stdNorm=eps  pSuccessGeo=40  meanPoiss=40  thresholdLogn=40  scaleLogn=40  shapeLogn=40  thresholdLogl=40  scaleLogl=40  minBeta=40  maxBeta=40  shape1Beta=40  shape2Beta=40  minUnid=40  maxUnid=40  numValueUnid=40  thresholdWbl=40  scaleWbl=40  shapeWbl=40  valueVecCont=40  cdfVecCont=40  valueVecDisc=40  probVecDisc=40  Seed=56120
  RandomNumbers_ProcessingTimes : EventBasedRandomNumber  meanExp=80  minUnif=40  maxUnif=40  pOneBern=40  pSuccessBino=40  numTrialBino=40  minTri=40  maxTri=40  modeTri=40  thresholdGam=40  scaleGam=40  shapeGam=40  meanNorm=50  stdNorm=eps  pSuccessGeo=40  meanPoiss=40  thresholdLogn=40  scaleLogn=40  shapeLogn=40  thresholdLogl=40  scaleLogl=40  minBeta=40  maxBeta=40  shape1Beta=40  shape2Beta=40  minUnid=40  maxUnid=40  numValueUnid=40  thresholdWbl=40  scaleWbl=40  shapeWbl=40  valueVecCont=40  cdfVecCont=40  valueVecDisc=40  probVecDisc=40  Seed=59337
  RandomNumbers_SetupTimes : EventBasedRandomNumber  meanExp=400  minUnif=40  maxUnif=40  pOneBern=40  pSuccessBino=40  numTrialBino=40  minTri=38  maxTri=38  modeTri=38  scaleGam=20  meanNorm=200  stdNorm=eps  pSuccessGeo=40  meanPoiss=40  thresholdLogn=40  scaleLogn=40  shapeLogn=40  thresholdLogl=40  scaleLogl=40  minBeta=40  maxBeta=40  shape1Beta=40  shape2Beta=40  minUnid=40  maxUnid=40  numValueUnid=40  thresholdWbl=40  scaleWbl=40  shapeWbl=40  valueVecCont=40  cdfVecCont=40  probVecDisc=[0 1]  Seed=62554
  Arrivals : PMIOPort  Port=1  Side=Left
  Departures : PMIOPort  Port=2  Side=Right
  WIP_samples : Outport
  WIP_average : Outport  Port=2
  CT_samples : Outport  Port=3
  CT_average : Outport  Port=4
  TH_samples : Outport  Port=5
  TH_average : Outport  Port=6
  Util_average : Outport  Port=7
  Avail_average : Outport  Port=8
  wires:
  RandomNumbers_ProcessingTimes/1 -> GG1Workstation_RandomCountUntilNonpreempSetup/1(ProcessingTime)
  GG1Workstation_RandomCountUntilNonpreempSetup/2(nDepartures) -> ComputeWIP/2(nDepartures), ComputeTH/2(nDepartures)
  GG1Workstation_RandomCountUntilNonpreempSetup/3(CT_samples) -> CT_samples/1
  GG1Workstation_RandomCountUntilNonpreempSetup/4(CT_average) -> CT_average/1
  ComputeWIP/1(WIP_samples) -> WIP_samples/1
  ComputeWIP/2(WIP_average) -> WIP_average/1
  GG1Workstation_RandomCountUntilNonpreempSetup/1(nArrivals) -> ComputeWIP/1(nArrivals)
  Clock/1 -> ComputeWIP/3(CurrentTime), ComputeTH/1(CurrentTime), ComputeUandA/1(CurrentTime)
  ComputeTH/1(TH_average) -> TH_average/1
  ComputeTH/2(TH_samples) -> TH_samples/1
  RandomNumbers_CountUntilSetup/1 -> GG1Workstation_RandomCountUntilNonpreempSetup/2(CountUntilSetup)
  RandomNumbers_SetupTimes/1 -> GG1Workstation_RandomCountUntilNonpreempSetup/3(SetupTime)
  GG1Workstation_RandomCountUntilNonpreempSetup/7(nInFailServer) -> ComputeUandA/2(nInFailServer)
  GG1Workstation_RandomCountUntilNonpreempSetup/8(nInProcServer) -> ComputeUandA/3(nInProcServer)
  ComputeUandA/1(Util_average) -> Util_average/1
  ComputeUandA/2(Avail_average) -> Avail_average/1
  connections:
  GG1Workstation_RandomCountUntilNonpreempSetup/RConn1 -- Departures/RConn1
  Arrivals/RConn1 -- GG1Workstation_RandomCountUntilNonpreempSetup/LConn1

== system SingleWorkstationModelLibrary/GGkWorkstation ==
  note: % LICENSE: 3-clause "Revised" or "New" or "Modified" BSD License.
      | % Copyright (c) 2015, Georgia Institute of Technology.
      | % All rights reserved.
      | %
      | % Redistribution and use in source and binary forms, with or without
      | % modification, are permitted provided that the following conditions are met:
      | % * Redistributions of source code must retain the above copyright
      | % notice, this list of conditions and the following disclaimer.
      | % * Redistributions in binary form must reproduce the above copyright
      | % notice, this list of conditions and the following disclaimer in the
      | % documentation and/or other materials provided with the distribution.
      | % * Neither the name of the Georgia Institute of Technology nor the
      | % names of its contributors may be used to endorse or promote products
      | % derived from this software without specific prior written permission.
      | %
      | % THIS SOFTWARE IS PROVIDED BY THE COPYRIGHT HOLDERS AND CONTRIBUTORS "AS IS" AND
      | % ANY EXPRESS OR IMPLIED WARRANTIES, INCLUDING, BUT NOT LIMITED TO, THE IMPLIED
      | % WARRANTIES OF MERCHANTABILITY AND FITNESS FOR A PARTICULAR PURPOSE ARE
      | % DISCLAIMED. IN NO EVENT SHALL THE GEORGIA INSTITUTE OF TECHNOLOGY BE LIABLE FOR
      | % ANY DIRECT, INDIRECT, INCIDENTAL, SPECIAL, EXEMPLARY, OR CONSEQUENTIAL DAMAGES
      | % (INCLUDING, BUT NOT LIMITED TO, PROCUREMENT OF SUBSTITUTE GOODS OR SERVICES;
      | % LOSS OF USE, DATA, OR PROFITS; OR BUSINESS INTERRUPTION) HOWEVER CAUSED AND
      | % ON ANY THEORY OF LIABILITY, WHETHER IN CONTRACT, STRICT LIABILITY, OR TORT
      | % (INCLUDING NEGLIGENCE OR OTHERWISE) ARISING IN ANY WAY OUT OF THE USE OF THIS
      | % SOFTWARE, EVEN IF ADVISED OF THE POSSIBILITY OF SUCH DAMAGE.
  Clock : Clock
  ComputeTH : Subsystem
  ComputeWIP : Subsystem
  GGkWorkstation : Subsystem  mask{Capacity=Inf, NumberOfServers=1}
      mask prompts: Capacity "Queue Capacity:"; NumberOfServers "Number of Servers:"
      mask TypeOptions Capacity: FIFOQueue/Capacity
      mask TypeOptions NumberOfServers: N-Server/NumberOfServers
      mask DialogControl DescTextVar Prompt: Plain-vanilla GGk Workstation, with a FIFOQueue and N-Server
  RandomNumbers_ProcessingTimes : EventBasedRandomNumber  meanExp=90  minUnif=40  maxUnif=40  pOneBern=40  pSuccessBino=40  numTrialBino=40  minTri=40  maxTri=40  modeTri=40  thresholdGam=40  scaleGam=40  shapeGam=40  meanNorm=95  stdNorm=eps  pSuccessGeo=40  meanPoiss=40  thresholdLogn=40  scaleLogn=40  shapeLogn=40  thresholdLogl=40  scaleLogl=40  minBeta=40  maxBeta=40  shape1Beta=40  shape2Beta=40  minUnid=40  maxUnid=40  numValueUnid=40  thresholdWbl=40  scaleWbl=40  shapeWbl=40  valueVecCont=40  cdfVecCont=40  valueVecDisc=40  probVecDisc=40  Seed=50510
  Arrivals : PMIOPort  Port=1  Side=Left
  Departures : PMIOPort  Port=2  Side=Right
  WIP_samples : Outport
  WIP_average : Outport  Port=2
  CT_samples : Outport  Port=3
  CT_average : Outport  Port=4
  TH_samples : Outport  Port=5
  TH_average : Outport  Port=6
  Util_average : Outport  Port=7
  wires:
  RandomNumbers_ProcessingTimes/1 -> GGkWorkstation/1(ProcessingTimes)
  GGkWorkstation/5(Util_average) -> Util_average/1
  GGkWorkstation/2(nDepartures) -> ComputeTH/2(nDepartures), ComputeWIP/2(nDepartures)
  GGkWorkstation/3(CT_samples) -> CT_samples/1
  GGkWorkstation/4(CT_average) -> CT_average/1
  ComputeWIP/1(WIP_samples) -> WIP_samples/1
  ComputeWIP/2(WIP_average) -> WIP_average/1
  GGkWorkstation/1(nArrivals) -> ComputeWIP/1(nArrivals)
  Clock/1 -> ComputeWIP/3(CurrentTime), ComputeTH/1(CurrentTime)
  ComputeTH/1(TH_average) -> TH_average/1
  ComputeTH/2(TH_samples) -> TH_samples/1
  connections:
  GGkWorkstation/RConn1 -- Departures/RConn1
  Arrivals/RConn1 -- GGkWorkstation/LConn1
